simulink model "robust_tracking_integral_exact"  (R2020b)
settings: Solver=ode45  StartTime=0.0  StopTime=5  FixedStep=T/10  RelTol=1e-3
undefined symbols (not defined in the file or in its folder): A0, B0, Beq_hat, C0, ctrl, D0, daq, degs2rpm, denHwa, denHws, denKi, drv, GAMMA, gbox, H0, J0, Jeq_hat, Ke, Ki, mot, N_u, N_x, numHwa, numHws, numKi, PHI, rads2rpm, sens, step_size, T, tau_hat
settings Model: Creator=utente  LastModifiedBy=utente
settings DataIOCC: ReturnWorkspaceOutputs=off

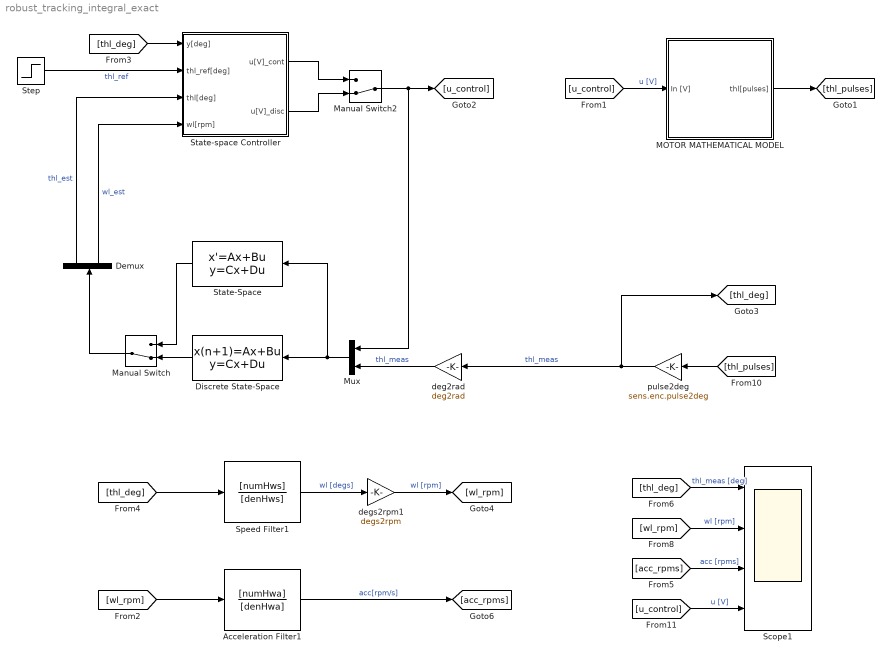
== system robust_tracking_integral_exact ==
  Acceleration Filter1 : TransferFcn  Numerator=[numHwa]  Denominator=[denHwa]
  Demux : Demux  Outputs=2
  Discrete State-Space : DiscreteStateSpace  A=PHI  B=GAMMA  C=H0  D=J0  SampleTime=T
  MOTOR MATHEMATICAL MODEL : Subsystem
  Manual Switch : ManualSwitch  CurrentSetting=0
  Manual Switch2 : ManualSwitch  CurrentSetting=0
  Mux : Mux  Inputs=2
  Scope1 : Scope  NumInputPorts=4
  Speed Filter1 : TransferFcn  Numerator=[numHws]  Denominator=[denHws]
  State-Space : StateSpace  A=A0  B=B0  C=C0  D=D0  InitialCondition=0
  State-space Controller : Subsystem
  Step : Step  After=step_size  SampleTime=0
  deg2rad : Gain  Gain=deg2rad
  degs2rpm1 : Gain  Gain=degs2rpm
  pulse2deg : Gain  Gain=sens.enc.pulse2deg
  wires:
  Step/1 -> State-space Controller/2(thl_ref[deg])  "thl_ref"
  pulse2deg/1 -> [thl_deg], deg2rad/1  "thl_meas"
  Mux/1 -> State-Space/1, Discrete State-Space/1
  Demux/1 -> State-space Controller/3(thl[deg])  "thl_est"
  State-Space/1 -> Manual Switch/1
  deg2rad/1 -> Mux/2  "thl_meas"
  Demux/2 -> State-space Controller/4(wl[rpm])  "wl_est"
  Manual Switch/1 -> Demux/1
  Discrete State-Space/1 -> Manual Switch/2
  [thl_deg] -> State-space Controller/1(y[deg])
  State-space Controller/1(u[V]_cont) -> Manual Switch2/1
  State-space Controller/2(u[V]_disc) -> Manual Switch2/2
  Manual Switch2/1 -> [u_control], Mux/1
  [u_control] -> MOTOR MATHEMATICAL MODEL/1(In [V])  "u [V]"
  MOTOR MATHEMATICAL MODEL/1(thl[pulses]) -> [thl_pulses]
  [thl_pulses] -> pulse2deg/1
  [thl_deg] -> Scope1/1  "thl_meas [deg]"
  [wl_rpm] -> Scope1/2  "wl [rpm]"
  [acc_rpms] -> Scope1/3  "acc [rpms]"
  [u_control] -> Scope1/4  "u [V]"
  [wl_rpm] -> Acceleration Filter1/1
  Speed Filter1/1 -> degs2rpm1/1  "wl [degs]"
  Acceleration Filter1/1 -> [acc_rpms]  "acc[rpm/s]"
  [thl_deg] -> Speed Filter1/1
  degs2rpm1/1 -> [wl_rpm]  "wl [rpm]"

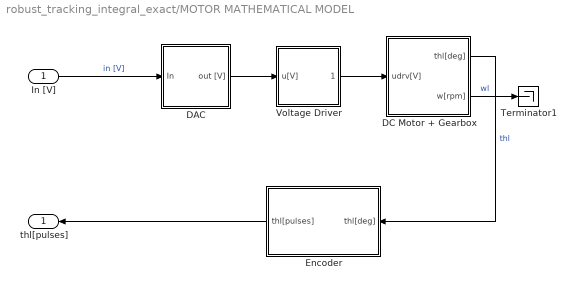
== system robust_tracking_integral_exact/MOTOR MATHEMATICAL MODEL ==
  In [V] : Inport
  DAC : Subsystem
  DC Motor + Gearbox : Subsystem
  Encoder : Subsystem
  Terminator1 : Terminator
  Voltage Driver : Subsystem
  thl[pulses] : Outport
  wires:
  Voltage Driver/1(udrv[V]) -> DC Motor + Gearbox/1(udrv[V])
  Encoder/1(thl[pulses]) -> thl[pulses]/1
  DC Motor + Gearbox/2(w[rpm]) -> Terminator1/1  "wl"
  DAC/1(out [V]) -> Voltage Driver/1(u[V])
  DC Motor + Gearbox/1(thl[deg]) -> Encoder/1(thl[deg])  "thl"
  In [V]/1 -> DAC/1(In)  "in [V]"

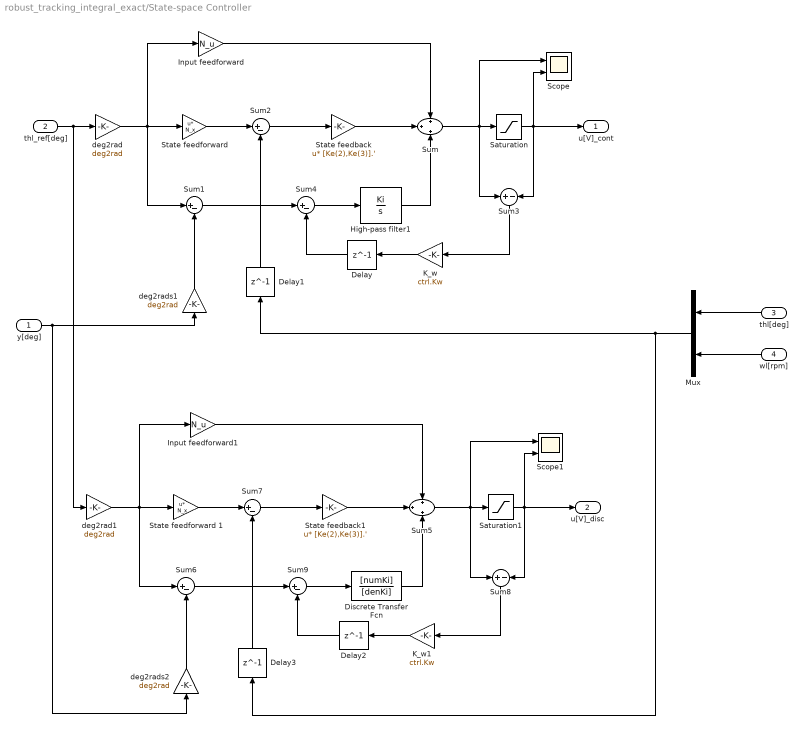
== system robust_tracking_integral_exact/State-space Controller ==
  y[deg] : Inport
  thl_ref[deg] : Inport  Port=2
  thl[deg] : Inport  Port=3
  wl[rpm] : Inport  Port=4
  Delay{,1..3} (4 alike) : Delay  DelayLength=1  InitialCondition=0
  Discrete Transfer Fcn : DiscreteTransferFcn  Numerator=[numKi]  Denominator=[denKi]  SampleTime=T
  High-pass filter1 : TransferFcn  Numerator=Ki  Denominator=[1 0]
  Input feedforward : Gain  Gain=N_u
  Input feedforward1 : Gain  Gain=N_u
  K_w : Gain  Gain=ctrl.Kw
  K_w1 : Gain  Gain=ctrl.Kw
  Mux : Mux  Inputs=2
  Saturation : Saturate  UpperLimit=10  LowerLimit=-10
  Saturation1 : Saturate  UpperLimit=10  LowerLimit=-10
  Scope : Scope  NumInputPorts=2
  Scope1 : Scope  NumInputPorts=2
  State feedback : Gain  Gain=[Ke(2),Ke(3)].'  Multiplication=Matrix(u*K)
  State feedback1 : Gain  Gain=[Ke(2),Ke(3)].'  Multiplication=Matrix(u*K)
  "State feedforward\t" : Gain  Gain=N_x  Multiplication=Matrix(u*K)
  State feedforward	1 : Gain  Gain=N_x  Multiplication=Matrix(u*K)
  Sum : Sum  Inputs=+|+|+
  Sum{1..2,4,6..7,9} (6 alike) : Sum  Inputs=|+-
  Sum3 : Sum  Inputs=+|-
  Sum5 : Sum  Inputs=+|+|+
  Sum8 : Sum  Inputs=+|-
  deg2rad : Gain  Gain=deg2rad
  deg2rad1 : Gain  Gain=deg2rad
  deg2rads1 : Gain  Gain=deg2rad
  deg2rads2 : Gain  Gain=deg2rad
  u[V]_cont : Outport
  u[V]_disc : Outport  Port=2
  wires:
  deg2rad/1 -> Sum1/1, Input feedforward/1, "State feedforward\t"/1
  State feedback/1 -> Sum/2
  "State feedforward\t"/1 -> Sum2/1
  Sum2/1 -> State feedback/1
  Input feedforward/1 -> Sum/1
  thl[deg]/1 -> Mux/1
  wl[rpm]/1 -> Mux/2
  Mux/1 -> Delay1/1, Delay3/1
  High-pass filter1/1 -> Sum/3
  Sum1/1 -> Sum4/1
  deg2rads1/1 -> Sum1/2
  Saturation/1 -> Sum3/2, Scope/2, u[V]_cont/1
  Sum3/1 -> K_w/1
  Sum/1 -> Sum3/1, Scope/1, Saturation/1
  Sum4/1 -> High-pass filter1/1
  K_w/1 -> Delay/1
  Delay/1 -> Sum4/2
  Delay1/1 -> Sum2/2
  Sum8/1 -> K_w1/1
  Sum9/1 -> Discrete Transfer Fcn/1
  y[deg]/1 -> deg2rads1/1, deg2rads2/1
  deg2rads2/1 -> Sum6/2
  K_w1/1 -> Delay2/1
  Sum5/1 -> Sum8/1, Scope1/1, Saturation1/1
  Sum6/1 -> Sum9/1
  Saturation1/1 -> Sum8/2, Scope1/2, u[V]_disc/1
  Input feedforward1/1 -> Sum5/1
  Delay2/1 -> Sum9/2
  State feedforward	1/1 -> Sum7/1
  State feedback1/1 -> Sum5/2
  Sum7/1 -> State feedback1/1
  deg2rad1/1 -> Sum6/1, Input feedforward1/1, State feedforward	1/1
  thl_ref[deg]/1 -> deg2rad1/1, deg2rad/1
  Delay3/1 -> Sum7/2
  Discrete Transfer Fcn/1 -> Sum5/3

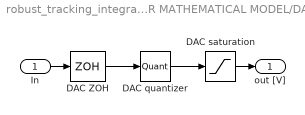
== system robust_tracking_integral_exact/MOTOR MATHEMATICAL MODEL/DAC ==
  In : Inport
  DAC quantizer : Quantizer  QuantizationInterval=daq.dac.q
  DAC saturation : Saturate  UpperLimit=daq.dac.fs  LowerLimit=-daq.dac.fs
  DAC ZOH : ZeroOrderHold  SampleTime=0.001
  out [V] : Outport
  wires:
  DAC ZOH/1 -> DAC quantizer/1
  DAC quantizer/1 -> DAC saturation/1
  In/1 -> DAC ZOH/1
  DAC saturation/1 -> out [V]/1

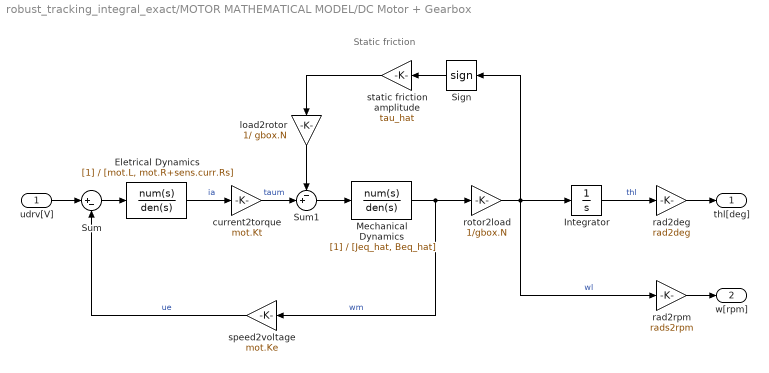
== system robust_tracking_integral_exact/MOTOR MATHEMATICAL MODEL/DC Motor + Gearbox ==
  note: Static friction
  udrv[V] : Inport
  Eletrical Dynamics : TransferFcn  Denominator=[mot.L, mot.R+sens.curr.Rs]
  Integrator : Integrator
  Mechanical Dynamics : TransferFcn  Denominator=[Jeq_hat, Beq_hat]
  Sign : Signum  ZeroCross=off
  Sum : Sum  Inputs=|+-
  Sum1 : Sum  Inputs=-+|
  current2torque : Gain  Gain=mot.Kt
  load2rotor : Gain  Gain=1/ gbox.N
  rad2deg : Gain  Gain=rad2deg
  "rad2rpm " : Gain  Gain=rads2rpm
  rotor2load : Gain  Gain=1/gbox.N
  speed2voltage : Gain  Gain=mot.Ke
  static friction amplitude : Gain  Gain=tau_hat
  thl[deg] : Outport  VectorParamsAs1DForOutWhenUnconnected=off
  w[rpm] : Outport  Port=2  VectorParamsAs1DForOutWhenUnconnected=off
  wires:
  Eletrical Dynamics/1 -> current2torque/1  "ia"
  udrv[V]/1 -> Sum/1
  Sum/1 -> Eletrical Dynamics/1
  current2torque/1 -> Sum1/2  "taum"
  Sum1/1 -> Mechanical Dynamics/1
  Mechanical Dynamics/1 -> rotor2load/1, speed2voltage/1  "wm"
  rotor2load/1 -> Integrator/1, "rad2rpm "/1, Sign/1  "wl"
  Integrator/1 -> rad2deg/1  "thl"
  rad2deg/1 -> thl[deg]/1
  "rad2rpm "/1 -> w[rpm]/1
  static friction amplitude/1 -> load2rotor/1
  Sign/1 -> static friction amplitude/1
  speed2voltage/1 -> Sum/2  "ue"
  load2rotor/1 -> Sum1/1

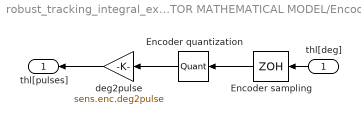
== system robust_tracking_integral_exact/MOTOR MATHEMATICAL MODEL/Encoder ==
  thl[deg] : Inport
  Encoder quantization : Quantizer  QuantizationInterval=sens.enc.pulse2deg
  Encoder sampling : ZeroOrderHold  SampleTime=-1
  deg2pulse : Gain  Gain=sens.enc.deg2pulse
  thl[pulses] : Outport
  wires:
  thl[deg]/1 -> Encoder sampling/1
  Encoder quantization/1 -> deg2pulse/1
  Encoder sampling/1 -> Encoder quantization/1
  deg2pulse/1 -> thl[pulses]/1

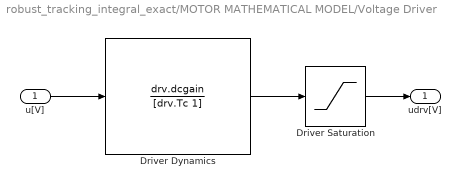
== system robust_tracking_integral_exact/MOTOR MATHEMATICAL MODEL/Voltage Driver ==
  u[V] : Inport
  Driver Dynamics : TransferFcn  Numerator=drv.dcgain  Denominator=[drv.Tc 1]
  Driver Saturation : Saturate  UpperLimit=12  LowerLimit=-12
  udrv[V] : Outport
  wires:
  Driver Dynamics/1 -> Driver Saturation/1
  Driver Saturation/1 -> udrv[V]/1
  u[V]/1 -> Driver Dynamics/1
